simulink model "prob_5"  (R2020b)
settings: Solver=VariableStepAuto  StartTime=0.0  StopTime=10.0  RelTol=1e-3
libraries: simulink x1
settings Model: Creator=Yeshwanth  LastModifiedBy=Yeshwanth

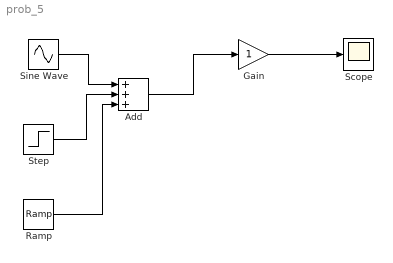
== system prob_5 ==
  Add : Sum  Inputs=+++
  Gain : Gain
  Ramp : simulink/Sources/Ramp  slope=1  start=0  InitialOutput=0
  Scope : Scope
  Sine Wave : Sin  SampleTime=0
  Step : Step  SampleTime=0
  wires:
  Gain/1 -> Scope/1
  Sine Wave/1 -> Add/1
  Step/1 -> Add/2
  Add/1 -> Gain/1
  Ramp/1 -> Add/3
